simulink library "dspcelplib"  (Simulink 6.0)
libraries: dspsrcs4 x1, dspindex x1
settings Model: Creator=The MathWorks Inc.  LastModifiedBy=batserve  ExtModeAutoUpdateStatusClock=off

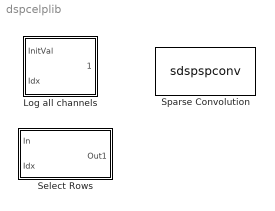
== system dspcelplib ==
  Log all channels : Subsystem  mask{outType=Row vector, numRow=40, numCol=4, dType=double}
      mask prompts: outType "Output type:"; numRow "Number of rows:"; numCol "Number of columns:"; dType "Data type:"
      mask init:
      | str = dspblklogdata('init');
      mask StyleString: popup(Row vector|Column vector|Matrix),edit,edit,popup(double|int32)
      mask CallbackString: dspblklogdata;|||
      mask Display:
      | port_label('input',1,'Val');
      | port_label('input',2,str);
      | port_label('output',1,'Out');
  Select Rows : Subsystem  mask(Select Rows){numRows=40}
      mask prompts: numRows "Number of rows (Nr):"
      mask help: Select a number of rows. The row indices are determined by the input index, Idx, and the total number of rows specified in the mask. The selected row indices are Idx, Idx+1, Idx+2, ..., Idx +Nr-1.
      mask init:
      | blk=gcb;
      | const_blk = [blk,'/SequenceGenerator/DSPConstant'];
      | numROWS = get_param(blk,'numRows');
      | 
      | val = ['[0:(',numROWS,'-1)]' ];
      | dspsafe_set_param(const_blk, 'Value', val);
  Sparse Convolution : S-Function  FunctionName=sdspspconv
      mask Type: Sparse Convolution
      mask Description: Convolve vectors A and B, where A is sparse and has an implicit full length of 40. Enter the sign of the nonzero elements of A at input port PA. Enter the zero-based indices of the nonzero elements of A at input port IA. The vectors input to ports PA and IA must have length 4. The vector input to port B must have length 40. The length of the output vector is 40. This block only supports frame-based signals.
      mask Help: web(dspbhelp);
      mask Display:
      | disp('Sparse\nConv');
      | port_label('input',1, 'PA');
      | port_label('input',2, 'IA');
      | port_label('input',3, 'B');
      | 
      | port_label('output',1, 'Out');

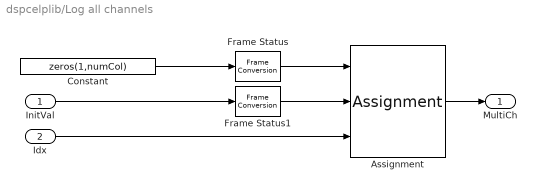
== system dspcelplib/Log all channels ==
  InitVal : Inport  Port=1  LatchInput=off
  Idx : Inport  Port=2  LatchInput=off
  Assignment : Assignment  ElementSrc=External  Rows=-1  ColumnSrc=External
  Constant : Constant  Value=zeros(1,numCol)  VectorParams1D=off  OutDataTypeMode=double
  Frame Status : FrameConversion
  Frame Status1 : FrameConversion
  MultiCh : Outport
  wires:
  Constant/1 -> Frame Status/1
  Frame Status/1 -> Assignment/1
  InitVal/1 -> Frame Status1/1
  Idx/1 -> Assignment/3
  Assignment/1 -> MultiCh/1
  Frame Status1/1 -> Assignment/2

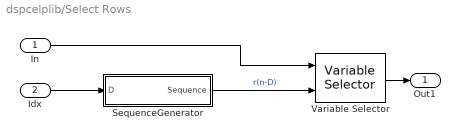
== system dspcelplib/Select Rows ==
  In : Inport  Port=1  LatchInput=off
  Idx : Inport  Port=2  LatchInput=off
  SequenceGenerator : Subsystem
  Variable Selector : dspindex/Variable Selector  rowsOrCols=Rows  IdxMode=Variable  Elements=[1 3]  ZerOneIdxMode=One-based  errmode=Generate Error
  Out1 : Outport
  wires:
  Idx/1 -> SequenceGenerator/1(D)
  Variable Selector/1 -> Out1/1
  In/1 -> Variable Selector/1
  SequenceGenerator/1(Sequence) -> Variable Selector/2  "r(n-D)"

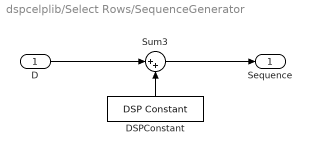
== system dspcelplib/Select Rows/SequenceGenerator ==
  D : Inport  Port=1  LatchInput=off
  DSPConstant : dspsrcs4/DSP Constant  Orientation=up  Value=[0:(numRows-1)]  SampleMode=Discrete  discreteOutput=Frame-based  continuousOutput=Sample-based  sampTime=1  framePeriod=-1  dataType=Inherit from 'Constant value'  isSigned=on  wordLen=16  udDataType=sfix(16)  fracBitsMode=Best precision  numFracBits=15  InterpretAs1D=-inf  Ts=-inf  FramebasedOutput=-inf
  Sum3 : Sum  Inputs=|++  SaturateOnIntegerOverflow=on
  Sequence : Outport
  wires:
  Sum3/1 -> Sequence/1
  D/1 -> Sum3/1
  DSPConstant/1 -> Sum3/2
